simulink model "closeLoopS"  (R2013b)
settings: Solver=ode1  StartTime=0.0  StopTime=tSim  FixedStep=0.1  RelTol=1e-3
undefined symbols (not defined in the file): initial_state, input, k, P, T
settings Model: Creator=JT  LastModifiedBy=JT

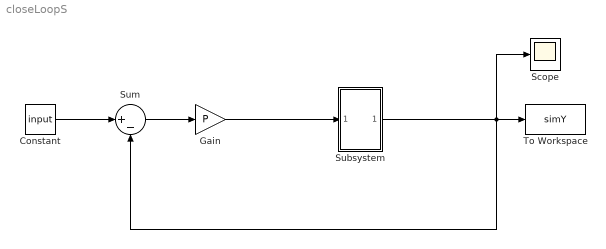
== system closeLoopS ==
  Constant : Constant  Value=input
  Gain : Gain  Gain=P
  Scope : Scope
  Subsystem : Subsystem
  Sum : Sum  Inputs=|+-
  To Workspace : ToWorkspace  VariableName=simY  SampleTime=-1
  wires:
  Constant/1 -> Sum/1
  Sum/1 -> Gain/1
  Gain/1 -> Subsystem/1(In1)
  Subsystem/1(Out1) -> Sum/2, Scope/1, To Workspace/1

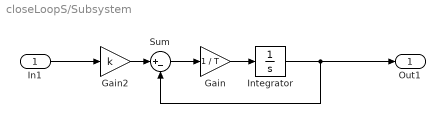
== system closeLoopS/Subsystem ==
  In1 : Inport
  Gain : Gain  Gain=1 / T
  Gain2 : Gain  Gain=k
  Integrator : Integrator  InitialCondition=initial_state
  Sum : Sum  Inputs=|+-
  Out1 : Outport
  wires:
  Sum/1 -> Gain/1
  Integrator/1 -> Out1/1, Sum/2
  Gain2/1 -> Sum/1
  In1/1 -> Gain2/1
  Gain/1 -> Integrator/1
